simulink model "Sender"  (R2021b)
settings: Solver=ode1  StartTime=0.0  StopTime=inf  FixedStep=0.001  RelTol=1e-3
undefined symbols (not defined in the file): delayTimeCarToDamper
settings Model: Creator=jalfonso  LastModifiedBy=au602135
settings SolverCC: AlgebraicLoopSolver=TrustRegion
settings DataIOCC: ReturnWorkspaceOutputs=off
settings DebuggingCC: SFMachineParentedDataDiag=warning  ArithmeticOperatorsInVariantConditions=warning
settings SFSimCC: SimUseLocalCustomCode=off  CustomCodeUndefinedFunction=UseInterfaceOnly
settings RTWCC: RTWUseLocalCustomCode=off
settings CodeAppCC: StateflowObjectComments=on

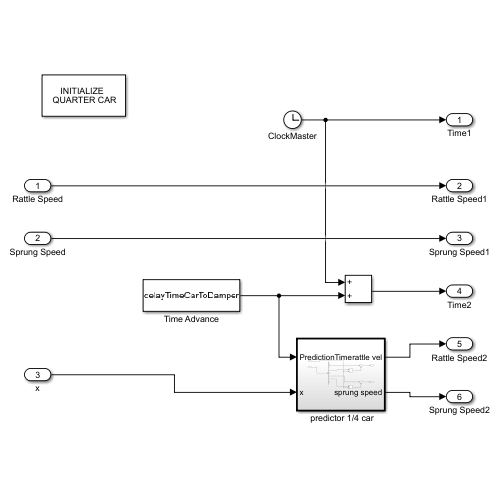
[thumbnail: Simulink's stored preview of the top-level diagram]
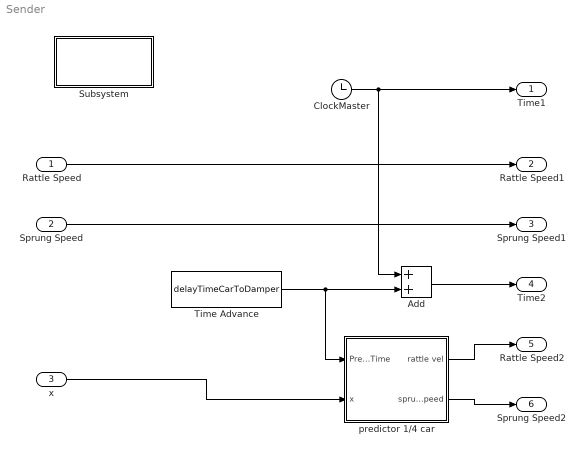
== system Sender ==
  Rattle Speed : Inport
  Sprung Speed : Inport  Port=2
  x : Inport  Port=3
  " predictor 1/4 car" : Subsystem  TreatAsAtomicUnit=on
  Add : Sum
  ClockMaster : Clock
  Subsystem : Subsystem
      settings: OpenFcn=|
      | k_tire = 225400;  %200000 in literature
      | c_tire = 100;        % Estimated. In literatures 6N
      | k_susp =  25000;  % 15000 in literature
      | c_susp = 400;       %1429 Ns/m in literature
      | g = 0 % 9.8; Removed to avoid initialization problems
      | m_unsprung = 66;
      | m_sprung = 449.25;
      | X_sprung0  = .5;
      | X_unsprung0  = .1;
      | delayTimeCarToDamper =  0.002;
      | %InitQuarterCarCompensatorScript;
      | %Amplitude =.01;
      mask Display: disp('INITIALIZE \n QUARTER CAR')
  Time Advance : Constant  Value=delayTimeCarToDamper
  Time1 : Outport
  Rattle Speed1 : Outport  Port=2
  Sprung Speed1 : Outport  Port=3
  Time2 : Outport  Port=4
  Rattle Speed2 : Outport  Port=5
  Sprung Speed2 : Outport  Port=6
  wires:
  Rattle Speed/1 -> Rattle Speed1/1
  Sprung Speed/1 -> Sprung Speed1/1
  " predictor 1/4 car"/1(rattle vel) -> Rattle Speed2/1
  Time Advance/1 -> " predictor 1/4 car"/1(PredictionTime), Add/2
  ClockMaster/1 -> Time1/1, Add/1
  Add/1 -> Time2/1
  x/1 -> " predictor 1/4 car"/2(x)
  " predictor 1/4 car"/2(sprung speed) -> Sprung Speed2/1

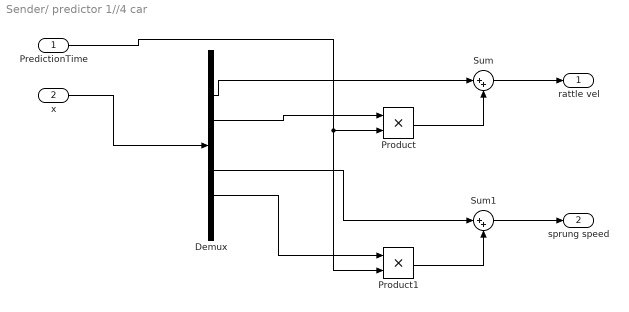
== system Sender/ predictor 1//4 car ==
  PredictionTime : Inport
  x : Inport  Port=2
  Demux : Demux  Outputs=7
  Product : Product
  Product1 : Product
  Sum : Sum  Inputs=|++
  Sum1 : Sum  Inputs=|++
  rattle vel : Outport
  sprung speed : Outport  Port=2
  wires:
  PredictionTime/1 -> Product1/2, Product/2
  x/1 -> Demux/1
  Demux/2 -> Sum/1
  Demux/3 -> Product/1
  Product/1 -> Sum/2
  Sum/1 -> rattle vel/1
  Demux/5 -> Sum1/1
  Product1/1 -> Sum1/2
  Sum1/1 -> sprung speed/1
  Demux/6 -> Product1/1

== system Sender/Subsystem ==
